simulink model "d_flip_flop"  (R2025b)
settings: Solver=VariableStepAuto  StartTime=0.0  StopTime=10.0  RelTol=1e-3
libraries: simulink_extras x1
settings Model: Creator=Johan  LastModifiedBy=Johan

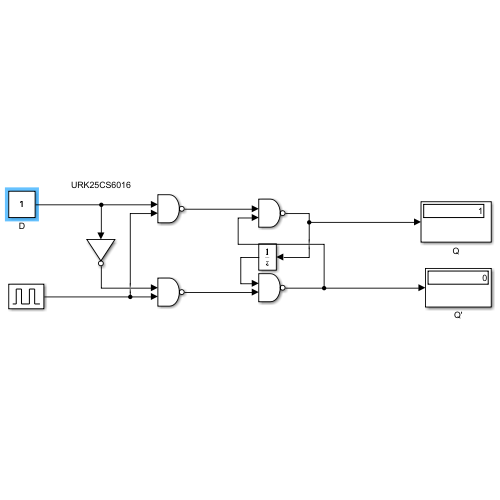
[thumbnail: Simulink's stored preview of the top-level diagram]
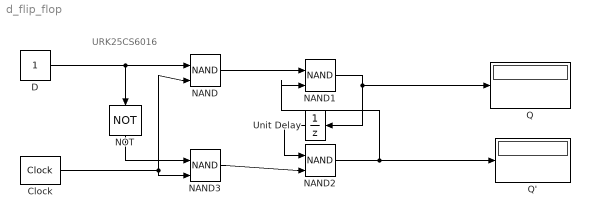
== system d_flip_flop ==
  note: URK25CS6016
  Clock : simulink_extras/Flip Flops/Clock  period=2
  D : Constant
  NAND{,1..3} (4 alike) : Logic  Operator=NAND  IconShape=distinctive  AllPortsSameDT=off  OutDataTypeStr=boolean
  NOT : Logic  Operator=NOT  IconShape=distinctive  AllPortsSameDT=off  OutDataTypeStr=boolean
  Q : Display
  Q' : Display
  Unit Delay : UnitDelay  SampleTime=-1  HasFrameUpgradeWarning=on
  wires:
  D/1 -> NOT/1, NAND/1
  NOT/1 -> NAND3/1
  Clock/1 -> NAND/2, NAND3/2
  NAND/1 -> NAND1/1
  NAND3/1 -> NAND2/2
  NAND2/1 -> NAND1/2, Q'/1
  NAND1/1 -> Unit Delay/1, Q/1
  Unit Delay/1 -> NAND2/1
